simulink model "punto_11"  (R2015a)
settings: Solver=ode45  StartTime=0.0  StopTime=100  RelTol=1e-3
values from neighbouring files (symbols this model uses):
  a = [-6 -11 -6;1 0 0;0 1 0]    [punto_1.m]    (also in punto_2.m = [0 1 0;0 0 1;-5 -6 0]; punto_3.m = [0 1 0;0 0 1;-1.244 -0.3956 -3.145]; punto_4.m = [0 1;0 0])
  b = [1;0;0]    [punto_1.m]    (also in punto_2.m = [0;0;1]; punto_3.m = [0;0;1.244]; punto_4.m = [0;1])
  c = [0 0 10]    [punto_1.m]    (also in punto_2.m = [1 0 0]; punto_3.m = [1 0 0]; punto_4.m = [1 0])
  d = 0    [punto_1.m]    (also in punto_2.m; punto_3.m; punto_4.m)
  k = place(a,b,p)    [punto_1.m]    (also in punto_2.m = acker(a,b,p); punto_3.m = place(a,b,p1); punto_4.m = place(a,b,prealim))
settings Model: Creator=Jose Roldan  LastModifiedBy=Jose Roldan

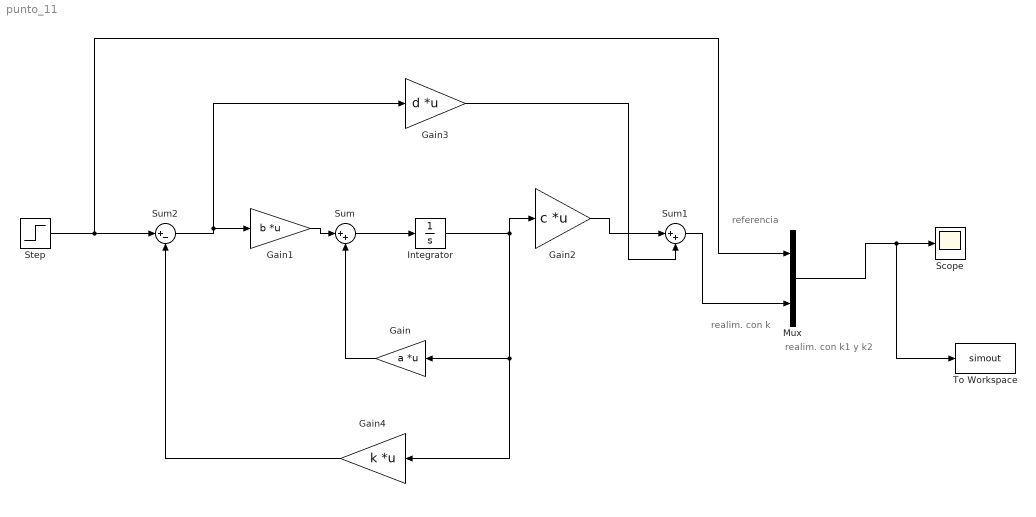
== system punto_11 ==
  note: realim. con k1 y k2
  note: realim. con k
  note: referencia
  Gain : Gain  Gain=a  Multiplication=Matrix(K*u)
  Gain1 : Gain  Gain=b  Multiplication=Matrix(K*u)
  Gain2 : Gain  Gain=c  Multiplication=Matrix(K*u)
  Gain3 : Gain  Gain=d  Multiplication=Matrix(K*u)
  Gain4 : Gain  Gain=k  Multiplication=Matrix(K*u)
  Integrator : Integrator
  Mux : Mux  Inputs=2
  Scope : Scope
  Step : Step  SampleTime=0
  Sum : Sum  Inputs=|++
  Sum1 : Sum  Inputs=|++
  Sum2 : Sum  Inputs=|+-
  To Workspace : ToWorkspace  VariableName=simout  SaveFormat=Timeseries  SampleTime=-1
  wires:
  Step/1 -> Mux/1, Sum2/1
  Sum2/1 -> Gain3/1, Gain1/1
  Gain1/1 -> Sum/1
  Sum/1 -> Integrator/1
  Integrator/1 -> Gain4/1, Gain/1, Gain2/1
  Gain2/1 -> Sum1/1
  Gain3/1 -> Sum1/2
  Gain/1 -> Sum/2
  Gain4/1 -> Sum2/2
  Sum1/1 -> Mux/2
  Mux/1 -> To Workspace/1, Scope/1
